simulink model "usrp_1t12r_heatmap"  (R2017b)
settings: Solver=VariableStepAuto  StartTime=0.0  StopTime=inf  RelTol=1e-3
undefined symbols (not defined in the file): get, parula, Time, us
libraries: dspsnks4 x6, commsdrhw_v2 x1, dspfdesign x1, dspstat3 x1, visiontransforms x1, visionanalysis x1, dspsigops x1, dspvision x1
settings Model: SimulationMode=accelerator  Creator=Sky  LastModifiedBy=Sky
settings DataIOCC: SaveTime=off
settings OptimizationCC: EfficientMapNaN2IntZero=off
settings HardwareCC: TargetBitPerPointer=64  TargetBitPerSizeT=64  TargetBitPerPtrDiffT=64  TargetLongLongMode=on  TargetIntDivRoundTo=Zero  TargetEndianess=LittleEndian  TargetWordSize=64  TargetHWDeviceType=MATLAB Host  ProdEqTarget=off
settings CodeAppCC: MaxIdLength=128  StateflowObjectComments=on
settings GRTTargetCC: TargetLangStandard=C89/C90 (ANSI)  CombineOutputUpdateFcns=off  GRTInterface=on

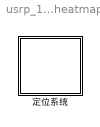
== system usrp_1t12r_heatmap ==
  定位系统 : Subsystem  mask{doSaveParam=on, decimInterp=100, fftDownFac=5, nCyclePF=4, fTr=800, tPul=0.1e-3, trThres=0, trEdge=0, antBits=logical(dec2bin(0:11)-48), antCoor=[[linspace(-0.053*(12/2-0.5),0.053*(12/2-0.5),12)',zeros(12,2)];0,0,-0.22], dMa=10, dMi=1, dCa=4.65+0.5, fCen=3.2e9, fBw=1e9, nAng=128, lFft=512}
      mask prompts: doSaveParam "save parameters to workspace"; decimInterp "decimation factor"; fftDownFac "fft downsample factor"; nCyclePF "cycles per frame (average time)"; fTr "triger frequency"; tPul "pulse time"; trThres "triger threshold"; trEdge "triger edge"; antBits "antenna bits"; antCoor "antenna coordinates"; dMa "distance max"; dMi "distance min"; dCa "cable length"; fCen "center frequency"; fBw "bandwidth"; nAng "angle FFT length"; lFft "dis FFT length"
      mask init:
      | global nRx lF fS lRamp nPul
      | nRx=size(antBits,1);
      | lF=100e6/decimInterp/fTr*nRx*nCyclePF;
      | fS=100e6/decimInterp;
      | lRamp=fS/fTr;%length ramp
      | nPul=size(antBits,2)+1;
      | 
      | global dLambda ds
      | dLambda=3e8/fCen;
      | fPm=fBw*fTr/3e8;%frequency per meter
      | fD=fS/fftDownFac/lFft;%frequency delta
      | fs=linspace(0,fS/fftDownFac/2-fD,floor(lFft/2));
      | ds=fs/fPm;
      | 
      | global angs
      | angMax=asind(dLambda/2/abs(antCoor(1,1)-antCoor(2,1)));
      | angs=linspace(-angMax,angMax,nAng);
      | 
      | % 排除线缆长度，截取有效距离
      | global dsC isD
      | dsC=(ds(ds>=dCa)-dCa)/2;
      | isD=find(dsC>=dMi & dsC<=dMa);
      | dsC=dsC(isD);
      | isD=isD+find(ds>=dCa,1)-1;
      | 
      | 
      | % 保存参数到工作空间base
      | if doSaveParam
      |     assignin('base','antBits',antBits);
      |     assignin('base','antCoor',antCoor);
      |     assignin('base','dMi',dMi);
      |     assignin('base','dMa',dMa);
      |     assignin('base','dCa',dCa);
      |     assignin('base','fS',fS);
      |     assignin('base','fTr',fTr);
      |     assignin('base','nCyclePF',nCyclePF);
      |     assignin('base','tPul',tPul);
      |     assignin('base','fCen',fCen);
      |     assignin('base','fBw',fBw);
      |     assignin('base','nAng',nAng);
      |     assignin('base','lFft',lFft);
      |     assignin('base','lRamp',lRamp);
      |     assignin('base','fftDownFac',fftDownFac);
      |     assignin('base','ds',ds);
      |     assignin('base','dsC',dsC);
      |     assignin('base','isD',isD);
      |     assignin('base','angs',angs);
      | end
      mask TypeOptions decimInterp: USRP/decimInterp
      mask Display: disp('定位系统');

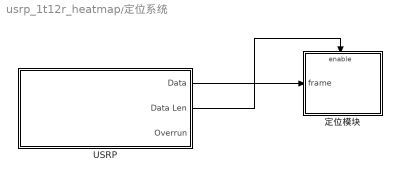
== system usrp_1t12r_heatmap/定位系统 ==
  USRP : Subsystem  mask{decimInterp=decimInterp, lF=lF}
      mask prompts: decimInterp "Decimation Factor"; lF "frameLength"
      mask TypeOptions decimInterp: SDRu Receiver/decimInterp
      mask TypeOptions lF: SDRu Receiver/frameLength
      mask Display: disp('USRP');
  定位模块 : Subsystem
  wires:
  USRP/1(Data) -> 定位模块/1(frame)
  USRP/2(Data Len) -> 定位模块/Enable

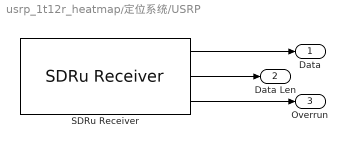
== system usrp_1t12r_heatmap/定位系统/USRP ==
  SDRu Receiver : commsdrhw_v2/SDRu Receiver  SourceLibraryInfo="This block requires <a href=\"http://www.mathworks.com/hardware-support/usrp.html\">Communications System Toolbox Support Package for USRP Radio</a>"  rxtx=rx  platform=N200/N210/USRP2  USRP2_IP='192.168.10.6'  USRP_IP_X300='192.168.10.2'  USRP_IP_X310='192.168.10.2'  USRP_serialNumB200=''  USRP_serialNumB210=''  ChannelMapping=1  centerFrequency=0  centerFrequencySrc=Dialog  loOffset=0  loOffsetSrc=Dialog  PPSSource=Internal  clockSource=Internal  masterClkRateB200=32e6  masterClkRateB210=32e6  masterClkRateX300=200e6  masterClkRateX310=200e6  masterClkRateParam=100e6  gain=0  gainSrc=Dialog  decimInterpSrc=Dialog  decimInterp=decimInterp  TransportDataType=int16  USRP2_IP_NUM=[49 57 50 46 49 54 56 46 49 48 46 54]  frameLength=lF  outputDatatype=single  overrunUnderrunPort=on  sampleTime=decimInterp/100e6  HOST_DATA_PORT=0  HOST_CONTROL_PORT=0  USRP2_DATA_PORT=0  USRP2_CONTROL_PORT=0  bufferMode=Continuous streaming  EnableBurstMode=off  NumFramesInBurst=10000  USRP_ID='192.168.10.6'
      settings: SourceProductName=Communications System Toolbox Support Package for USRP(R) Radio  SourceProductBaseCode=USRP
  Data : Outport
  Data Len : Outport  Port=2
  Overrun : Outport  Port=3
  wires:
  SDRu Receiver/2 -> Data Len/1
  SDRu Receiver/3 -> Overrun/1
  SDRu Receiver/1 -> Data/1

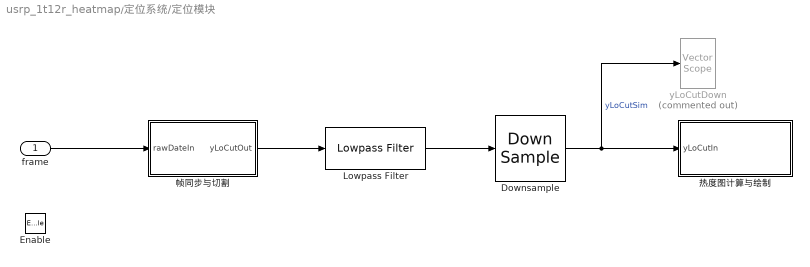
== system usrp_1t12r_heatmap/定位系统/定位模块 ==
  frame : Inport
  Enable : EnablePort
  Downsample : DownSample  N=fftDownFac
  Lowpass Filter : dspfdesign/Lowpass Filter  FilterType=FIR  DesignForMinimumOrder=off  FilterOrder=15  PassbandFrequency=fS/2/fftDownFac*0.8  StopbandFrequency=fS/2/fftDownFac  PassbandRipple=0.1  StopbandAttenuation=60  InheritSampleRate=off  SampleRate=fS  SimulateUsing=Code generation  roundingMode=Floor  coeffsDataTypeStr=fixdt(1,16)
  yLoCutDown : dspsnks4/Vector Scope  Commented=on  ScopeProperties=on  Domain=User-defined  HorizSpan=1  DisplayProperties=off  AxisGrid=on  Memory=off  FrameNumber=on  AxisLegend=off  AxisZoom=off  OpenScopeAtSimStart=on  OpenScopeImmediately=off  FigPos=get(0,'defaultfigureposition')  AxisProperties=off  XUnits=Hertz  XRange=[0...Fs/2]  InheritXIncr=off  XIncr=1e6/fS  XLabel=Time(us)  XLimit=Auto  XMin=0  XMax=1  XStart=0  YUnits=dB  YLabel=Amplitude  LineProperties=off  LineColors=[1 0 0]|[0 1 0]|[0 0 1]  XAxisParamsVer=6.9
      settings: SourceProductName=DSP System Toolbox  SourceProductBaseCode=DS  YMin=-0.3  YMax=0.3
  帧同步与切割 : Subsystem
  热度图计算与绘制 : Subsystem
  wires:
  frame/1 -> 帧同步与切割/1(rawDateIn)
  帧同步与切割/1(yLoCutOut) -> Lowpass Filter/1
  Downsample/1 -> yLoCutDown/1, 热度图计算与绘制/1(yLoCutIn)  "yLoCutSim"
  Lowpass Filter/1 -> Downsample/1

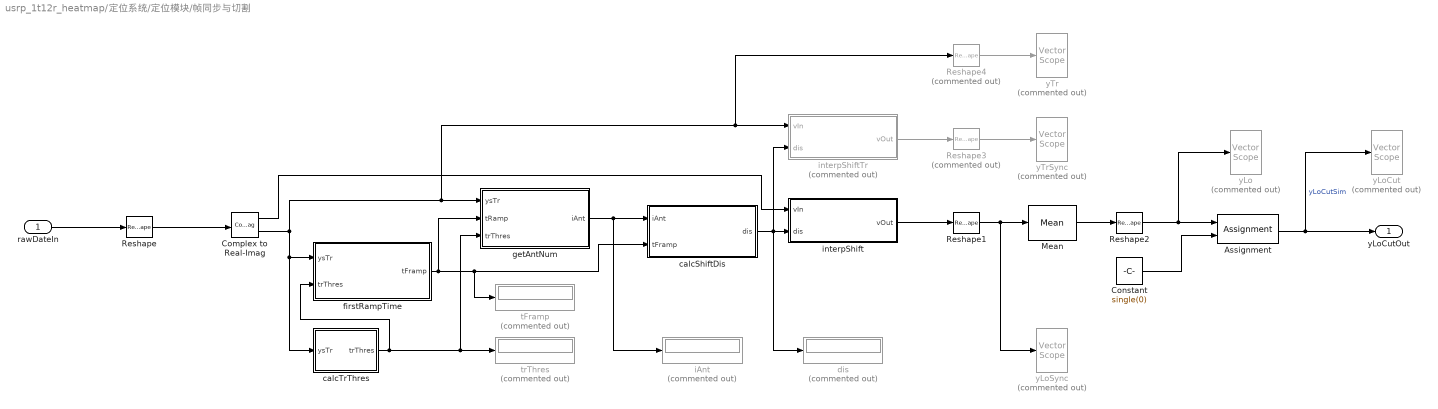
== system usrp_1t12r_heatmap/定位系统/定位模块/帧同步与切割 ==
  rawDateIn : Inport
  Assignment : Assignment  NumberOfDimensions=2  DiagnosticForDimensions=Warning  IndexOptions=Index vector (dialog),Assign all  Indices=[1:ceil(2e-5*fS),lRamp-ceil(2e-5*fS):lRamp],1  OutputSizes=1,1
  Complex to Real-Imag : ComplexToRealImag
  Constant : Constant  Value=single(0)
  Mean : dspstat3/Mean  run=off  reset_popup=None  InputProcessing=Columns as channels (frame based)  directionMode=Each row  dimension=1  roiEnable=off  roiType=Rectangles  roiPortion=Entire ROI  roiOutput=Individual statistics for each ROI  roiFlag=off  outputDataTypeStr=Inherit: Same as accumulator  outputLastDataTypeStr=Inherit: Same as accumulator  outputMin=[]  outputMax=[]  roundingMode=Floor  overflowMode=off
  Reshape : Reshape  OutputDimensionality=Row vector (2-D)
  Reshape1 : Reshape  OutputDimensionality=Customize  OutputDimensions=[lRamp*nRx,nCyclePF]
  Reshape2 : Reshape  OutputDimensionality=Customize  OutputDimensions=[lRamp,nRx]
  Reshape3 : Reshape  Commented=on  OutputDimensionality=Column vector (2-D)
  Reshape4 : Reshape  Commented=on  OutputDimensionality=Column vector (2-D)
  calcShiftDis : MATLAB Function  TreatAsAtomicUnit=on
  calcTrThres : MATLAB Function  TreatAsAtomicUnit=on
  dis : Display  Commented=on
  firstRampTime : MATLAB Function  TreatAsAtomicUnit=on
  getAntNum : MATLAB Function  TreatAsAtomicUnit=on
  iAnt : Display  Commented=on
  interpShift : MATLAB Function  TreatAsAtomicUnit=on
  interpShiftTr : MATLAB Function  Commented=on  TreatAsAtomicUnit=on
  tFramp : Display  Commented=on
  trThres : Display  Commented=on
  yLo : dspsnks4/Vector Scope  Commented=on  ScopeProperties=on  Domain=User-defined  HorizSpan=1  DisplayProperties=off  AxisGrid=on  Memory=off  FrameNumber=on  AxisLegend=off  AxisZoom=off  OpenScopeAtSimStart=on  OpenScopeImmediately=off  FigPos=get(0,'defaultfigureposition')  AxisProperties=off  XUnits=Hertz  XRange=[0...Fs/2]  InheritXIncr=off  XIncr=1e6/fS  XLabel=Time(us)  XLimit=Auto  XMin=0  XMax=1  XStart=0  YUnits=dB  YLabel=Amplitude  LineProperties=off  LineColors=[1 0 0]|[0 1 0]|[0 0 1]  XAxisParamsVer=6.9
      settings: SourceProductName=DSP System Toolbox  SourceProductBaseCode=DS  YMin=-0.3  YMax=0.3
  yLoCut : dspsnks4/Vector Scope  Commented=on  ScopeProperties=on  Domain=User-defined  HorizSpan=1  DisplayProperties=off  AxisGrid=on  Memory=off  FrameNumber=on  AxisLegend=off  AxisZoom=off  OpenScopeAtSimStart=on  OpenScopeImmediately=off  FigPos=get(0,'defaultfigureposition')  AxisProperties=off  XUnits=Hertz  XRange=[0...Fs/2]  InheritXIncr=off  XIncr=1e6/fS  XLabel=Time(us)  XLimit=Auto  XMin=0  XMax=1  XStart=0  YUnits=dB  YLabel=Amplitude  LineProperties=off  LineColors=[1 0 0]|[0 1 0]|[0 0 1]  XAxisParamsVer=6.9
      settings: SourceProductName=DSP System Toolbox  SourceProductBaseCode=DS  YMin=-0.3  YMax=0.3
  yLoSync : dspsnks4/Vector Scope  Commented=on  ScopeProperties=on  Domain=User-defined  HorizSpan=1  DisplayProperties=off  AxisGrid=on  Memory=off  FrameNumber=on  AxisLegend=off  AxisZoom=off  OpenScopeAtSimStart=on  OpenScopeImmediately=off  FigPos=get(0,'defaultfigureposition')  AxisProperties=off  XUnits=Hertz  XRange=[0...Fs/2]  InheritXIncr=off  XIncr=1e6/fS  XLabel=Time(us)  XLimit=Auto  XMin=0  XMax=1  XStart=0  YUnits=dB  YLabel=Amplitude  LineProperties=off  LineColors=[1 0 0]|[0 1 0]|[0 0 1]  XAxisParamsVer=6.9
      settings: SourceProductName=DSP System Toolbox  SourceProductBaseCode=DS  YMin=-0.3  YMax=0.3
  yTr : dspsnks4/Vector Scope  Commented=on  ScopeProperties=on  Domain=User-defined  HorizSpan=1  DisplayProperties=off  AxisGrid=on  Memory=off  FrameNumber=on  AxisLegend=off  AxisZoom=off  OpenScopeAtSimStart=on  OpenScopeImmediately=off  FigPos=get(0,'defaultfigureposition')  AxisProperties=off  XUnits=Hertz  XRange=[0...Fs/2]  InheritXIncr=off  XIncr=1e6/fS  XLabel=Time(us)  XLimit=Auto  XMin=0  XMax=1  XStart=0  YUnits=dB  YLabel=Amplitude  LineProperties=off  LineColors=[1 0 0]|[0 1 0]|[0 0 1]  XAxisParamsVer=6.9
      settings: SourceProductName=DSP System Toolbox  SourceProductBaseCode=DS  YMin=-0.6  YMax=0.2
  yTrSync : dspsnks4/Vector Scope  Commented=on  ScopeProperties=on  Domain=User-defined  HorizSpan=1  DisplayProperties=off  AxisGrid=on  Memory=off  FrameNumber=on  AxisLegend=off  AxisZoom=off  OpenScopeAtSimStart=on  OpenScopeImmediately=off  FigPos=get(0,'defaultfigureposition')  AxisProperties=off  XUnits=Hertz  XRange=[0...Fs/2]  InheritXIncr=off  XIncr=1e6/fS  XLabel=Time(us)  XLimit=Auto  XMin=0  XMax=1  XStart=0  YUnits=dB  YLabel=Amplitude  LineProperties=off  LineColors=[1 0 0]|[0 1 0]|[0 0 1]  XAxisParamsVer=6.9
      settings: SourceProductName=DSP System Toolbox  SourceProductBaseCode=DS  YMin=-0.6  YMax=0.2
  yLoCutOut : Outport
  wires:
  firstRampTime/1(tFramp) -> tFramp/1, calcShiftDis/2(tFramp), getAntNum/2(tRamp)
  getAntNum/1(iAnt) -> iAnt/1, calcShiftDis/1(iAnt)
  Complex to Real-Imag/1 -> interpShift/1(vIn)
  Reshape/1 -> Complex to Real-Imag/1
  interpShift/1(vOut) -> Reshape1/1
  Reshape2/1 -> yLo/1, Assignment/1
  calcTrThres/1(trThres) -> trThres/1, getAntNum/3(trThres), firstRampTime/2(trThres)
  Constant/1 -> Assignment/2
  calcShiftDis/1(dis) -> dis/1, interpShift/2(dis), interpShiftTr/2(dis)
  Mean/1 -> Reshape2/1
  rawDateIn/1 -> Reshape/1
  Assignment/1 -> yLoCutOut/1, yLoCut/1  "yLoCutSim"
  interpShiftTr/1(vOut) -> Reshape3/1
  Reshape3/1 -> yTrSync/1
  Complex to Real-Imag/2 -> calcTrThres/1(ysTr), firstRampTime/1(ysTr), Reshape4/1, interpShiftTr/1(vIn), getAntNum/1(ysTr)
  Reshape4/1 -> yTr/1
  Reshape1/1 -> yLoSync/1, Mean/1

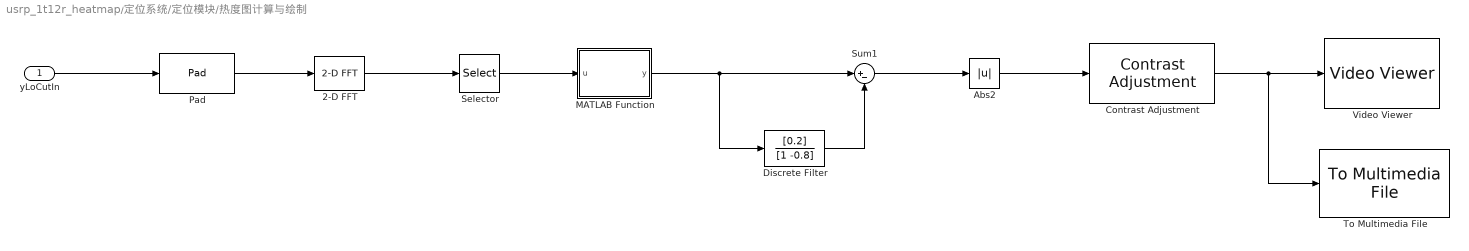
== system usrp_1t12r_heatmap/定位系统/定位模块/热度图计算与绘制 ==
  yLoCutIn : Inport
  2-D FFT : visiontransforms/2-D FFT  TableOpt=NEW  TableOptActive=Speed  BitRevOrder=off  SkipNorm=off  FFTImplementation=Auto  firstCoeffDataTypeStr=Inherit: Same word length as input  firstCoeffLastDataTypeStr=Inherit: Same word length as input  outputMin=[]  outputMax=[]  roundingMode=Floor  overflowMode=off
      settings: SourceProductName=Computer Vision System Toolbox  SourceProductBaseCode=VP
  Abs2 : Abs
  Contrast Adjustment : visionanalysis/Contrast Adjustment  methodInputRange=Full input data range [min max]  rangeIn=[0 255]  fracSaturate=[1 1]  isBinNum=on  binNum=256  methodOutputRange=Full data type range  rangeOut=[0 255]  prod1Mode=Binary point scaling  prod1WordLength=32  prod1FracLength=16  prod2Mode=Binary point scaling  prod2WordLength=32  prod2FracLength=16  roundingMode=Floor  overflowMode=off
      settings: SourceProductName=Computer Vision System Toolbox  SourceProductBaseCode=VP
  Discrete Filter : DiscreteFilter  Numerator=[0.2]  Denominator=[1 -0.8]
  MATLAB Function : MATLAB Function  TreatAsAtomicUnit=on
  Pad : dspsigops/Pad  padAlong=Columns and rows  dimsToPad=1  valSrc=Specify via dialog  padVal=0  spec=Output size  padNumOutRowsSpecMethod=User-specified  numOutRows=lFft  padNumOutColsSpecMethod=User-specified  numOutCols=nAng  isVarDimsMode=off  padBeginning=0  padEnd=0  outSizeMode=User-specified  outSize=1  padSigAt=End  trunc_flag=None  roundingMode=Floor  overflowMode=off  truncOrWrapMode=Truncate  wrap_flag=None
      settings: SourceProductName=DSP System Toolbox  SourceProductBaseCode=DS
  Selector : Selector  NumberOfDimensions=2  InputPortWidth=3  IndexOptions=Index vector (dialog),Select all  Indices=find(dsC>=dMi & dsC<=dMa)+find(ds>=dCa,1),1  OutputSizes=1,1
  Sum1 : Sum  Inputs=|+-
  To Multimedia File : dspvision/To Multimedia File  outputFilename=E:\Projects\2018_嵌入式邀请赛\FMCW定位系统\output.mp4  streamSelection=Video only  videoCompressor=None (uncompressed)  audioCompressor=None (uncompressed)  imagePorts=One multidimensional signal  fileType=MPEG4  audioDatatype=Determine from input data type  fourcc=RGB  videoQuality=75  mj2000CompFactor=10
      settings: SourceProductName=Computer Vision System Toolbox  SourceProductBaseCode=VP
  Video Viewer : VideoViewer  useColorMap=on  colormapValue=parula(256)  FigPos=[1141 729 418 304]
  wires:
  yLoCutIn/1 -> Pad/1
  Pad/1 -> 2-D FFT/1
  2-D FFT/1 -> Selector/1
  Discrete Filter/1 -> Sum1/2
  Sum1/1 -> Abs2/1
  Abs2/1 -> Contrast Adjustment/1
  MATLAB Function/1(y) -> Discrete Filter/1, Sum1/1
  Selector/1 -> MATLAB Function/1(u)
  Contrast Adjustment/1 -> To Multimedia File/1, Video Viewer/1

== matlab function usrp_1t12r_heatmap/定位系统/定位模块/帧同步与切割/getAntNum ==
  data: ysTr input; tRamp input; iAnt output; fS parameter; tPul parameter; antBits parameter; trThres input
%% 判断触发时间对应同步信号的天线编号
% iAnt: 天线编号
% ysTr: 一帧triger信号
% tRamp: 斜坡开始时间，以第一个采样点为参考时间0
% fS: 采样率
% tPul: 脉冲/比特宽度
% trThres: 触发电平
% antBits: 天线编号
function iAnt=getAntNum(ysTr, tRamp, fS, tPul, antBits, trThres)
if isnan(tRamp)
    iAnt=nan;
    return
end
%% 准备参数
lPul=fS*tPul;%length pulse

%% 抽取天线编号的比特电平
iBit1=ceil((tRamp+1.5*tPul)*fS)+1;
isBits=mod(linspace(iBit1,iBit1+lPul*(size(antBits,2)-1),size(antBits,2))-1,length(ysTr))+1;

ysBits=ysTr(isBits);
isAnt=find(all(~xor(antBits,repmat((ysBits>trThres),size(antBits,1),1)),2),1);
if isempty(isAnt)
    iAnt=nan;
    return
end
iAnt=isAnt(1);%为simulink推理iAnt大小提供帮助

end

== matlab function usrp_1t12r_heatmap/定位系统/定位模块/帧同步与切割/firstRampTime ==
  data: ysTr input; tFramp output; fS parameter; fTr parameter; tPul parameter; nPul parameter; trEdge parameter; trThres input; nRx parameter
%% 同步斜坡信号起始时间函数，返回所有斜坡信号起始时间点
% tFramp: 第一个斜坡开始时间，精确到采样时间之下，以第一个采样点为参考时间0
% ysTr: 一帧triger信号
% fS: 采样率
% fTr: 触发信号频率
% tPul: 脉冲/比特宽度
% nPul: 脉冲/比特总数
% trEdge: 触发沿：1上升沿 0下降沿
% trThres: 触发电平
function tFramp=firstRampTime(ysTr, fS, fTr, tPul, nPul, trEdge, trThres,nRx)
%% 准备参数
lRamp=fS/fTr;%length ramp
lPul=fS*tPul;%length pulse

if(mod(size(ysTr,2),lRamp)~=0)
    error('The length of frame is not integer multiple of the length of ramp .');
end

%% 分析第一个完整斜坡同步信号
%第一个完整斜坡同步信号触发沿位于1:lRamp,为了容错，扩大范围到1:lRamp+lPul*nPul
if(nRx>1)
    isFramp=1:lRamp+lPul*nPul;%indexs first ramp
else
    isFramp=1:lRamp;
end
ysTrFf=ysTr(isFramp);%ys triger first ramp
isTr=[];
if trEdge==0
    isTr=find(ysTrFf(2:end)<trThres & ysTrFf(1:end-1)>=trThres)+1;%index triger first
else
    isTr=find(ysTrFf(2:end)>trThres & ysTrFf(1:end-1)<=trThres)+1;
end
iTrF=0;
if isempty(isTr)
    tFramp=single(nan);
    return
else
    iTrF=isTr(find([true diff(isTr,1,2)>lPul*nPul],1,'last'));%要求脉冲和比特总时长小于斜坡周期的一半,选取最后一个触发信号
%     iTrF=isTrSync(end);
end


%% 线性插值分析上升沿的精确时间
tFramp=interp1([ysTr(iTrF-1),ysTr(iTrF)],([iTrF-1,iTrF]-1)/fS,trThres);
end

== matlab function usrp_1t12r_heatmap/定位系统/定位模块/帧同步与切割/interpShiftTr ==
  data: vIn input; vOut output; dis input
%% 循环移位，通过线性插值实现小数位数的移位
% vOut: 输出向量
% vIn: 输入向量
% dis: 向右移位距离
function vOut=interpShift(vIn, dis)
    if isnan(dis)
        vOut=vIn;
        return
    end
    isZeroBased=0:length(vIn)-1;
    if dis>=0
        iShift=floor(dis);
        iAdd=dis-iShift;
    else
        iShift=ceil(dis);
        iAdd=iShift-dis;
    end
    
    isShifted=circshift(isZeroBased,iShift);
    iInterp=isShifted+iAdd;
    vOut=interp1(isZeroBased,vIn,iInterp,'linear','extrap');
end

== matlab function usrp_1t12r_heatmap/定位系统/定位模块/帧同步与切割/calcShiftDis ==
  data: iAnt input; dis output; tFramp input; lRamp parameter; fS parameter; nRx parameter
%% 通过天线序号、时间偏移计算循环移位位移量
% dis: 位移量
% iAnt: 天线序号，从1开始
% tFramp: 第一个触发信号时间
% fS: 采样率
% nRx: 天线数量
function dis=calcShiftDis(iAnt,tFramp,lRamp,fS,nRx)
    dis=-((nRx+1-iAnt)*lRamp+(tFramp*fS));
end

== matlab function usrp_1t12r_heatmap/定位系统/定位模块/帧同步与切割/interpShift ==
  data: vIn input; vOut output; dis input
%% 循环移位，通过线性插值实现小数位数的移位
% vOut: 输出向量
% vIn: 输入向量
% dis: 向右移位距离
function vOut=interpShift(vIn, dis)
    if isnan(dis)
        vOut=vIn;
        return
    end
    isZeroBased=0:length(vIn)-1;
    if dis>=0
        iShift=floor(dis);
        iAdd=dis-iShift;
    else
        iShift=ceil(dis);
        iAdd=iShift-dis;
    end
    
    isShifted=circshift(isZeroBased,iShift);
    iInterp=isShifted+iAdd;
    vOut=interp1(isZeroBased,vIn,iInterp,'linear','extrap');
end

== matlab function usrp_1t12r_heatmap/定位系统/定位模块/帧同步与切割/calcTrThres ==
  data: ysTr input; trThres output
%% 计算触发电平
function trThres = calcTrThres(ysTr)
trThres=(max(ysTr)+min(ysTr))/2;%triger threshold
% trThres=(mean(ysTr(ysTr>trThres))+mean(ysTr(ysTr<trThres)))/2;
end

== matlab function usrp_1t12r_heatmap/定位系统/定位模块/热度图计算与绘制/MATLAB Function ==
  data: u input; y output
function y = heatMapShift(u)
y =circshift(u,ceil(size(u,2)/2),2);
